simulink model "Active_Rectifier"  (R2022b)
settings: Solver=VariableStepAuto  StartTime=0.0  StopTime=10.0  RelTol=1e-3
libraries: spsIGBTDiodeLib x6, spsSeriesRLCBranchLib x1
settings Model: Creator=Admin  LastModifiedBy=Admin

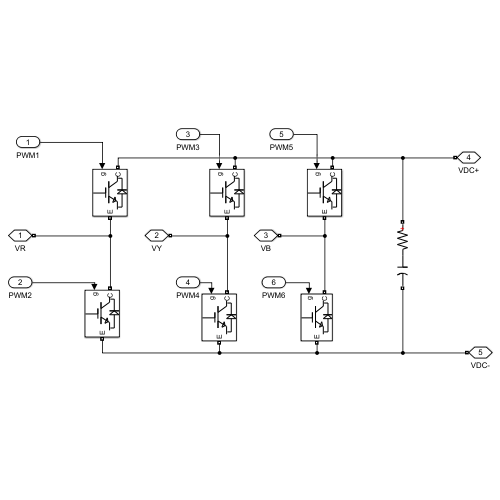
[thumbnail: Simulink's stored preview of the top-level diagram]
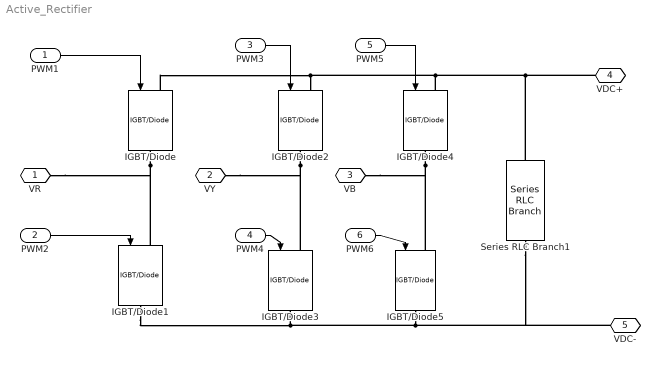
== system Active_Rectifier ==
  PWM1 : Inport
  PWM2 : Inport  Port=2
  PWM3 : Inport  Port=3
  PWM4 : Inport  Port=4
  PWM5 : Inport  Port=5
  PWM6 : Inport  Port=6
  IGBT/Diode{,1..5} (6 alike) : spsIGBTDiodeLib/IGBT//Diode  Ron=1e-3  Rs=1e5  Cs=inf  Measurements=off
  Series RLC Branch1 : spsSeriesRLCBranchLib/Series RLC Branch  LConnTagsString=__new0  RConnTagsString=__new0  BranchType=RC  Resistance=1e-3  Inductance=1e-3  SetiL0=off  InitialCurrent=0  Capacitance=5600e-6  Setx0=off  InitialVoltage=0  Measurements=None
  VR : PMIOPort  Side=Left
  VY : PMIOPort  Port=2  Side=Left
  VB : PMIOPort  Port=3  Side=Left
  VDC+ : PMIOPort  Port=4  Side=Right
  VDC- : PMIOPort  Port=5  Side=Right
  wires:
  PWM3/1 -> IGBT/Diode2/1
  PWM6/1 -> IGBT/Diode5/1
  PWM4/1 -> IGBT/Diode3/1
  PWM2/1 -> IGBT/Diode1/1
  PWM1/1 -> IGBT/Diode/1
  PWM5/1 -> IGBT/Diode4/1
  connections:
  Series RLC Branch1/LConn1 -- IGBT/Diode4/LConn1 -- IGBT/Diode/LConn1 -- IGBT/Diode2/LConn1 -- VDC+/RConn1
  IGBT/Diode2/RConn1 -- IGBT/Diode3/LConn1 -- VY/RConn1
  IGBT/Diode3/RConn1 -- IGBT/Diode5/RConn1 -- VDC-/RConn1 -- Series RLC Branch1/RConn1 -- IGBT/Diode1/RConn1
  IGBT/Diode4/RConn1 -- IGBT/Diode5/LConn1 -- VB/RConn1
  IGBT/Diode/RConn1 -- IGBT/Diode1/LConn1 -- VR/RConn1
